simulink model "with_extended_look_ahead"  (R2022a)
settings: Solver=FixedStepAuto  StartTime=0.0  StopTime=18  FixedStep=0.01  RelTol=1e-3
settings Model: Creator=11913  LastModifiedBy=11913

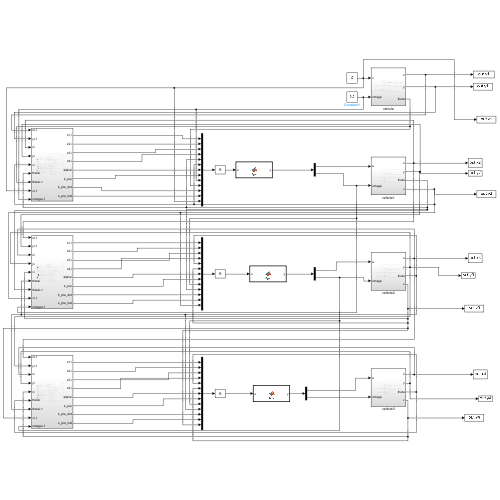
[thumbnail: Simulink's stored preview of the top-level diagram]
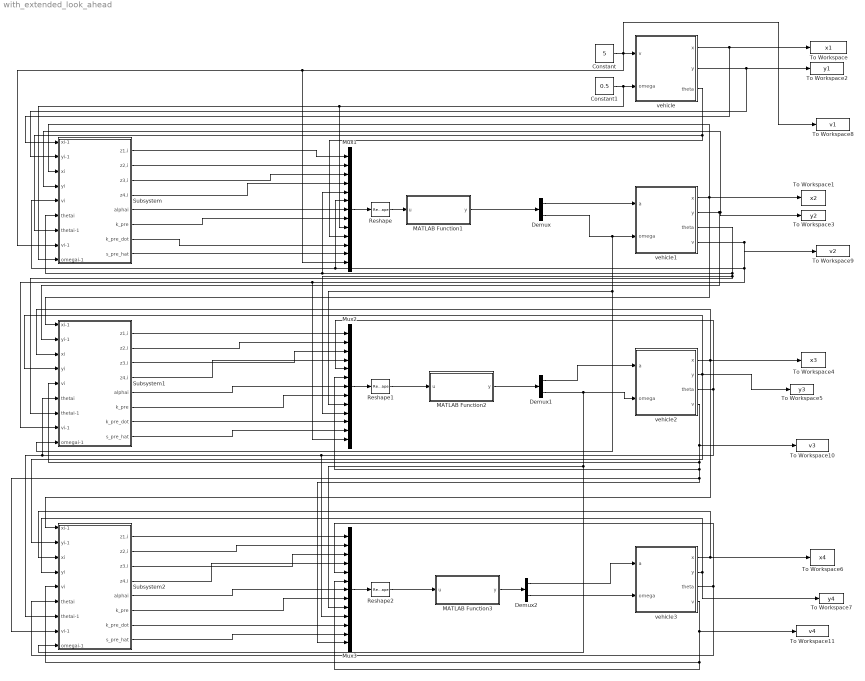
== system with_extended_look_ahead ==
  Constant : Constant  Value=5
  Constant1 : Constant  Value=0.5
  Demux : Demux  Outputs=2
  Demux1 : Demux  Outputs=2
  Demux2 : Demux  Outputs=2
  MATLAB Function1 : MATLAB Function  TreatAsAtomicUnit=on
  MATLAB Function2 : MATLAB Function  TreatAsAtomicUnit=on
  MATLAB Function3 : MATLAB Function  TreatAsAtomicUnit=on
  Mux1 : Mux  Inputs=13
  Mux2 : Mux  Inputs=13
  Mux3 : Mux  Inputs=13
  Reshape : Reshape  OutputDimensionality=Customize  OutputDimensions=[1,13]
  Reshape1 : Reshape  OutputDimensionality=Customize  OutputDimensions=[1,13]
  Reshape2 : Reshape  OutputDimensionality=Customize  OutputDimensions=[1,13]
  Subsystem : Subsystem
  Subsystem1 : Subsystem
  Subsystem2 : Subsystem
  To Workspace : ToWorkspace  VariableName=x1  SampleTime=-1
      settings: Save2DSignal=2-D array (concatenate along first dimension)
  To Workspace1 : ToWorkspace  VariableName=x2  SampleTime=-1
      settings: Save2DSignal=2-D array (concatenate along first dimension)
  To Workspace10 : ToWorkspace  VariableName=v3  SaveFormat=Timeseries  SampleTime=-1
      settings: Save2DSignal=2-D array (concatenate along first dimension)
  To Workspace11 : ToWorkspace  VariableName=v4  SaveFormat=Timeseries  SampleTime=-1
      settings: Save2DSignal=2-D array (concatenate along first dimension)
  To Workspace2 : ToWorkspace  VariableName=y1  SampleTime=-1
      settings: Save2DSignal=2-D array (concatenate along first dimension)
  To Workspace3 : ToWorkspace  VariableName=y2  SampleTime=-1
      settings: Save2DSignal=2-D array (concatenate along first dimension)
  To Workspace4 : ToWorkspace  VariableName=x3  SampleTime=-1
      settings: Save2DSignal=2-D array (concatenate along first dimension)
  To Workspace5 : ToWorkspace  VariableName=y3  SampleTime=-1
      settings: Save2DSignal=2-D array (concatenate along first dimension)
  To Workspace6 : ToWorkspace  VariableName=x4  SampleTime=-1
      settings: Save2DSignal=2-D array (concatenate along first dimension)
  To Workspace7 : ToWorkspace  VariableName=y4  SampleTime=-1
      settings: Save2DSignal=2-D array (concatenate along first dimension)
  To Workspace8 : ToWorkspace  VariableName=v1  SaveFormat=Timeseries  SampleTime=-1
      settings: Save2DSignal=2-D array (concatenate along first dimension)
  To Workspace9 : ToWorkspace  VariableName=v2  SaveFormat=Timeseries  SampleTime=-1
      settings: Save2DSignal=2-D array (concatenate along first dimension)
  vehicle : Subsystem
  vehicle1 : Subsystem
  vehicle2 : Subsystem
  vehicle3 : Subsystem
  wires:
  Constant/1 -> To Workspace8/1, Mux1/13, Subsystem/8(vi-1), vehicle/1(v)
  Constant1/1 -> Subsystem/9(omegai-1), Mux1/9, vehicle/2(omega)
  vehicle/2(y) -> To Workspace2/1, Subsystem/2(yi-1)
  vehicle/1(x) -> To Workspace/1, Subsystem/1(xi-1)
  vehicle/3(theta) -> Mux1/10, Subsystem/7(thetai-1)
  vehicle1/1(x) -> Subsystem1/1(xi-1), Subsystem/3(xi), To Workspace1/1
  vehicle1/2(y) -> Subsystem1/2(yi-1), To Workspace3/1, Subsystem/4(yi)
  vehicle1/4(v) -> To Workspace9/1, Mux2/13, Subsystem1/8(vi-1), Subsystem/5(vi), Mux1/6
  vehicle1/3(theta) -> Mux2/10, Subsystem1/7(thetai-1), Subsystem/6(thetai), Mux1/5
  Subsystem/1(z1,i) -> Mux1/1
  Subsystem/2(z2,i) -> Mux1/2
  Subsystem/3(z3,i) -> Mux1/3
  Subsystem/4(z4,i) -> Mux1/4
  Subsystem/5(alphai) -> Mux1/7
  Subsystem/6(k_pre) -> Mux1/8
  Subsystem/7(k_pre_dot) -> Mux1/11
  Subsystem/8(s_pre_hat) -> Mux1/12
  MATLAB Function1/1(y) -> Demux/1
  Demux/1 -> vehicle1/1(a)
  Demux/2 -> Mux2/9, Subsystem1/9(omegai-1), vehicle1/2(omega)
  Mux1/1 -> Reshape/1
  Reshape/1 -> MATLAB Function1/1(u)
  vehicle2/1(x) -> Subsystem2/1(xi-1), To Workspace4/1, Subsystem1/3(xi)
  vehicle2/2(y) -> Subsystem2/2(yi-1), To Workspace5/1, Subsystem1/4(yi)
  vehicle2/4(v) -> To Workspace10/1, Mux3/13, Subsystem2/8(vi-1), Mux2/6, Subsystem1/5(vi)
  vehicle2/3(theta) -> Mux3/10, Subsystem2/7(thetai-1), Subsystem1/6(thetai), Mux2/5
  Subsystem1/1(z1,i) -> Mux2/1
  Subsystem1/2(z2,i) -> Mux2/2
  Subsystem1/3(z3,i) -> Mux2/3
  Subsystem1/4(z4,i) -> Mux2/4
  Subsystem1/5(alphai) -> Mux2/7
  Subsystem1/6(k_pre) -> Mux2/8
  Subsystem1/7(k_pre_dot) -> Mux2/11
  Subsystem1/8(s_pre_hat) -> Mux2/12
  Mux2/1 -> Reshape1/1
  Reshape1/1 -> MATLAB Function2/1(u)
  MATLAB Function2/1(y) -> Demux1/1
  Demux1/1 -> vehicle2/1(a)
  Demux1/2 -> Mux3/9, Subsystem2/9(omegai-1), vehicle2/2(omega)
  vehicle3/1(x) -> To Workspace6/1, Subsystem2/3(xi)
  vehicle3/2(y) -> To Workspace7/1, Subsystem2/4(yi)
  vehicle3/4(v) -> Mux3/6, Subsystem2/5(vi), To Workspace11/1
  vehicle3/3(theta) -> Subsystem2/6(thetai), Mux3/5
  Subsystem2/1(z1,i) -> Mux3/1
  Subsystem2/2(z2,i) -> Mux3/2
  Subsystem2/3(z3,i) -> Mux3/3
  Subsystem2/4(z4,i) -> Mux3/4
  Subsystem2/5(alphai) -> Mux3/7
  Subsystem2/6(k_pre) -> Mux3/8
  Subsystem2/7(k_pre_dot) -> Mux3/11
  Subsystem2/8(s_pre_hat) -> Mux3/12
  Mux3/1 -> Reshape2/1
  Reshape2/1 -> MATLAB Function3/1(u)
  MATLAB Function3/1(y) -> Demux2/1
  Demux2/1 -> vehicle3/1(a)
  Demux2/2 -> vehicle3/2(omega)

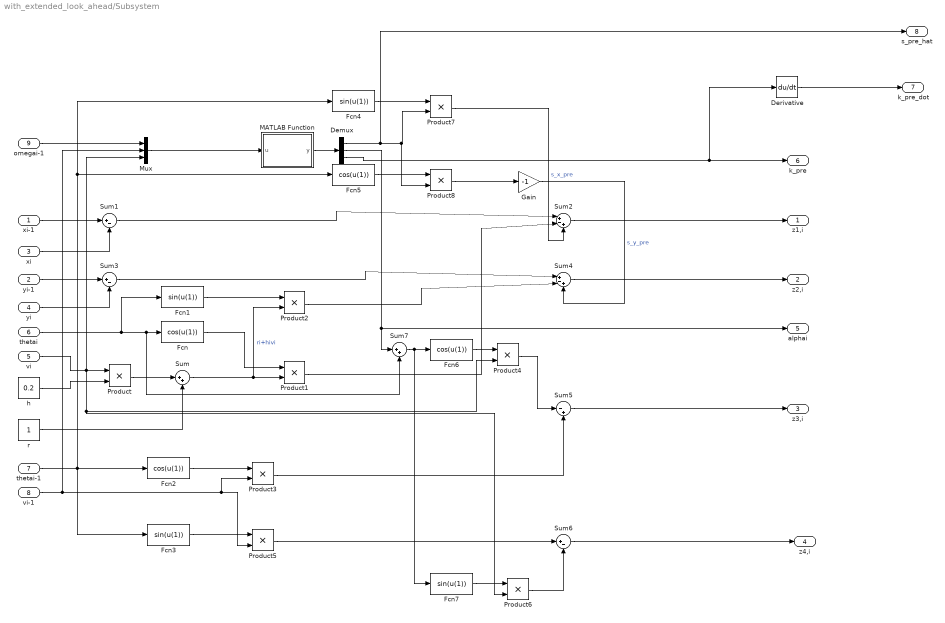
== system with_extended_look_ahead/Subsystem ==
  xi-1 : Inport
  yi-1 : Inport  Port=2
  xi : Inport  Port=3
  yi : Inport  Port=4
  vi : Inport  Port=5
  thetai : Inport  Port=6
  thetai-1 : Inport  Port=7
  vi-1 : Inport  Port=8
  omegai-1 : Inport  Port=9
  Demux : Demux  Outputs=3
  Derivative : Derivative
  Fcn{,2,5..6} (4 alike) : Fcn  Expr=cos(u(1))
  Fcn{1,3..4,7} (4 alike) : Fcn  Expr=sin(u(1))
  Gain : Gain  Gain=-1
  MATLAB Function : MATLAB Function  TreatAsAtomicUnit=on
  Mux : Mux  Inputs=3
  Product{,1..8} (9 alike) : Product
  Sum : Sum  Inputs=|++
  Sum1 : Sum  Inputs=|+-
  Sum2 : Sum  Inputs=|+-+
  Sum3 : Sum  Inputs=|+-
  Sum4 : Sum  Inputs=|+-+
  Sum5 : Sum  Inputs=|-+
  Sum6 : Sum  Inputs=|+-
  Sum7 : Sum  Inputs=|++
  h : Constant  Value=0.2
  r : Constant
  z1,i : Outport
  z2,i : Outport  Port=2
  z3,i : Outport  Port=3
  z4,i : Outport  Port=4
  alphai : Outport  Port=5
  k_pre : Outport  Port=6
  k_pre_dot : Outport  Port=7
  s_pre_hat : Outport  Port=8
  wires:
  vi/1 -> Product6/2, Product4/2, Mux/3, Product/1
  h/1 -> Product/2
  Product/1 -> Sum/1
  r/1 -> Sum/2
  xi-1/1 -> Sum1/1
  xi/1 -> Sum1/2
  thetai/1 -> Sum7/2, Fcn/1, Fcn1/1
  Sum/1 -> Product2/2, Product1/2  "ri+hivi"
  Fcn/1 -> Product1/1
  Sum1/1 -> Sum2/1
  Product1/1 -> Sum2/2
  yi-1/1 -> Sum3/1
  yi/1 -> Sum3/2
  Fcn1/1 -> Product2/1
  Sum3/1 -> Sum4/1
  Product2/1 -> Sum4/2
  Sum4/1 -> z2,i/1
  Sum2/1 -> z1,i/1
  thetai-1/1 -> Fcn5/1, Fcn4/1, Fcn3/1, Fcn2/1
  Fcn2/1 -> Product3/1
  vi-1/1 -> Mux/2, Product5/2, Product3/2
  Product3/1 -> Sum5/2
  Sum5/1 -> z3,i/1
  Fcn3/1 -> Product5/1
  Product5/1 -> Sum6/1
  Sum6/1 -> z4,i/1
  omegai-1/1 -> Mux/1
  Mux/1 -> MATLAB Function/1(u)
  Fcn4/1 -> Product7/1
  Product7/1 -> Sum2/3  "s_x_pre"
  Fcn5/1 -> Product8/1
  Product8/1 -> Gain/1
  Gain/1 -> Sum4/3  "s_y_pre"
  MATLAB Function/1(y) -> Demux/1
  Demux/1 -> s_pre_hat/1, Product8/2, Product7/2
  Demux/2 -> alphai/1, Sum7/1
  Sum7/1 -> Fcn7/1, Fcn6/1
  Fcn6/1 -> Product4/1
  Product4/1 -> Sum5/1
  Fcn7/1 -> Product6/1
  Product6/1 -> Sum6/2
  Demux/3 -> Derivative/1, k_pre/1
  Derivative/1 -> k_pre_dot/1

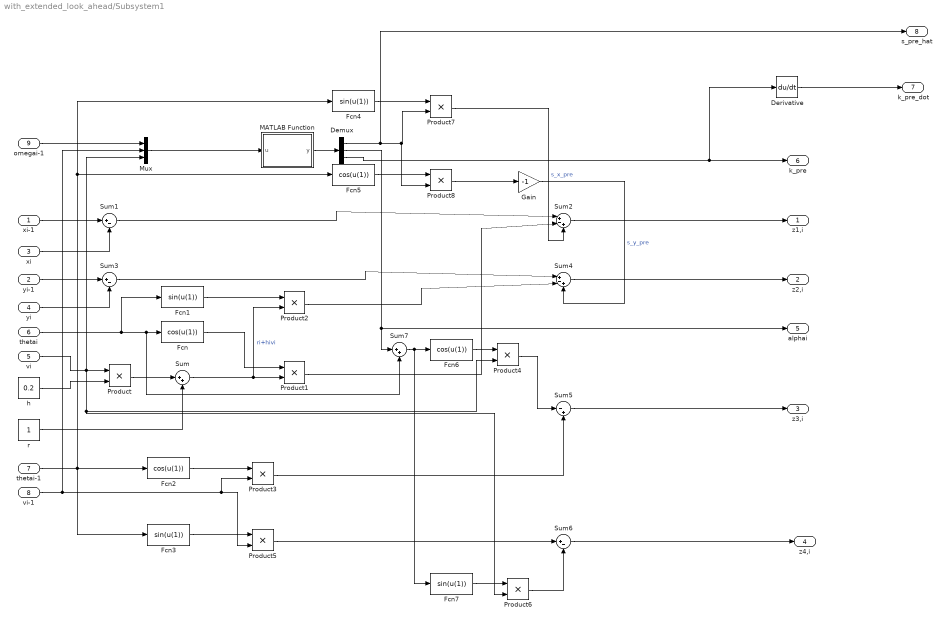
== system with_extended_look_ahead/Subsystem1 ==
  xi-1 : Inport
  yi-1 : Inport  Port=2
  xi : Inport  Port=3
  yi : Inport  Port=4
  vi : Inport  Port=5
  thetai : Inport  Port=6
  thetai-1 : Inport  Port=7
  vi-1 : Inport  Port=8
  omegai-1 : Inport  Port=9
  Demux : Demux  Outputs=3
  Derivative : Derivative
  Fcn{,2,5..6} (4 alike) : Fcn  Expr=cos(u(1))
  Fcn{1,3..4,7} (4 alike) : Fcn  Expr=sin(u(1))
  Gain : Gain  Gain=-1
  MATLAB Function : MATLAB Function  TreatAsAtomicUnit=on
  Mux : Mux  Inputs=3
  Product{,1..8} (9 alike) : Product
  Sum : Sum  Inputs=|++
  Sum1 : Sum  Inputs=|+-
  Sum2 : Sum  Inputs=|+-+
  Sum3 : Sum  Inputs=|+-
  Sum4 : Sum  Inputs=|+-+
  Sum5 : Sum  Inputs=|-+
  Sum6 : Sum  Inputs=|+-
  Sum7 : Sum  Inputs=|++
  h : Constant  Value=0.2
  r : Constant
  z1,i : Outport
  z2,i : Outport  Port=2
  z3,i : Outport  Port=3
  z4,i : Outport  Port=4
  alphai : Outport  Port=5
  k_pre : Outport  Port=6
  k_pre_dot : Outport  Port=7
  s_pre_hat : Outport  Port=8
  wires:
  vi/1 -> Product6/2, Product4/2, Mux/3, Product/1
  h/1 -> Product/2
  Product/1 -> Sum/1
  r/1 -> Sum/2
  xi-1/1 -> Sum1/1
  xi/1 -> Sum1/2
  thetai/1 -> Sum7/2, Fcn/1, Fcn1/1
  Sum/1 -> Product2/2, Product1/2  "ri+hivi"
  Fcn/1 -> Product1/1
  Sum1/1 -> Sum2/1
  Product1/1 -> Sum2/2
  yi-1/1 -> Sum3/1
  yi/1 -> Sum3/2
  Fcn1/1 -> Product2/1
  Sum3/1 -> Sum4/1
  Product2/1 -> Sum4/2
  Sum4/1 -> z2,i/1
  Sum2/1 -> z1,i/1
  thetai-1/1 -> Fcn5/1, Fcn4/1, Fcn3/1, Fcn2/1
  Fcn2/1 -> Product3/1
  vi-1/1 -> Mux/2, Product5/2, Product3/2
  Product3/1 -> Sum5/2
  Sum5/1 -> z3,i/1
  Fcn3/1 -> Product5/1
  Product5/1 -> Sum6/1
  Sum6/1 -> z4,i/1
  omegai-1/1 -> Mux/1
  Mux/1 -> MATLAB Function/1(u)
  Fcn4/1 -> Product7/1
  Product7/1 -> Sum2/3  "s_x_pre"
  Fcn5/1 -> Product8/1
  Product8/1 -> Gain/1
  Gain/1 -> Sum4/3  "s_y_pre"
  MATLAB Function/1(y) -> Demux/1
  Demux/1 -> s_pre_hat/1, Product8/2, Product7/2
  Demux/2 -> alphai/1, Sum7/1
  Sum7/1 -> Fcn7/1, Fcn6/1
  Fcn6/1 -> Product4/1
  Product4/1 -> Sum5/1
  Fcn7/1 -> Product6/1
  Product6/1 -> Sum6/2
  Demux/3 -> Derivative/1, k_pre/1
  Derivative/1 -> k_pre_dot/1

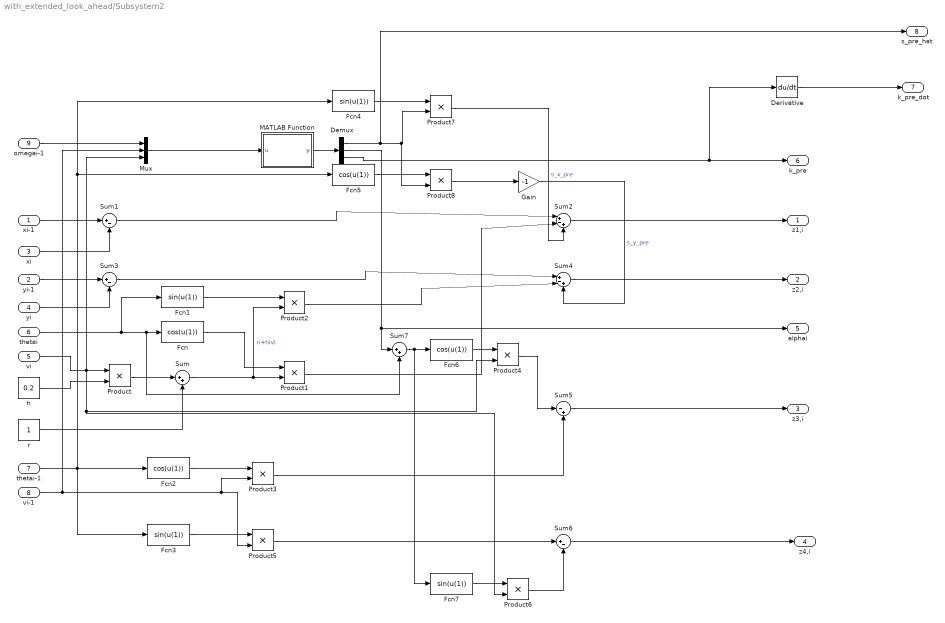
== system with_extended_look_ahead/Subsystem2 ==
  xi-1 : Inport
  yi-1 : Inport  Port=2
  xi : Inport  Port=3
  yi : Inport  Port=4
  vi : Inport  Port=5
  thetai : Inport  Port=6
  thetai-1 : Inport  Port=7
  vi-1 : Inport  Port=8
  omegai-1 : Inport  Port=9
  Demux : Demux  Outputs=3
  Derivative : Derivative
  Fcn{,2,5..6} (4 alike) : Fcn  Expr=cos(u(1))
  Fcn{1,3..4,7} (4 alike) : Fcn  Expr=sin(u(1))
  Gain : Gain  Gain=-1
  MATLAB Function : MATLAB Function  TreatAsAtomicUnit=on
  Mux : Mux  Inputs=3
  Product{,1..8} (9 alike) : Product
  Sum : Sum  Inputs=|++
  Sum1 : Sum  Inputs=|+-
  Sum2 : Sum  Inputs=|+-+
  Sum3 : Sum  Inputs=|+-
  Sum4 : Sum  Inputs=|+-+
  Sum5 : Sum  Inputs=|-+
  Sum6 : Sum  Inputs=|+-
  Sum7 : Sum  Inputs=|++
  h : Constant  Value=0.2
  r : Constant
  z1,i : Outport
  z2,i : Outport  Port=2
  z3,i : Outport  Port=3
  z4,i : Outport  Port=4
  alphai : Outport  Port=5
  k_pre : Outport  Port=6
  k_pre_dot : Outport  Port=7
  s_pre_hat : Outport  Port=8
  wires:
  vi/1 -> Product6/2, Product4/2, Mux/3, Product/1
  h/1 -> Product/2
  Product/1 -> Sum/1
  r/1 -> Sum/2
  xi-1/1 -> Sum1/1
  xi/1 -> Sum1/2
  thetai/1 -> Sum7/2, Fcn/1, Fcn1/1
  Sum/1 -> Product2/2, Product1/2  "ri+hivi"
  Fcn/1 -> Product1/1
  Sum1/1 -> Sum2/1
  Product1/1 -> Sum2/2
  yi-1/1 -> Sum3/1
  yi/1 -> Sum3/2
  Fcn1/1 -> Product2/1
  Sum3/1 -> Sum4/1
  Product2/1 -> Sum4/2
  Sum4/1 -> z2,i/1
  Sum2/1 -> z1,i/1
  thetai-1/1 -> Fcn5/1, Fcn4/1, Fcn3/1, Fcn2/1
  Fcn2/1 -> Product3/1
  vi-1/1 -> Mux/2, Product5/2, Product3/2
  Product3/1 -> Sum5/2
  Sum5/1 -> z3,i/1
  Fcn3/1 -> Product5/1
  Product5/1 -> Sum6/1
  Sum6/1 -> z4,i/1
  omegai-1/1 -> Mux/1
  Mux/1 -> MATLAB Function/1(u)
  Fcn4/1 -> Product7/1
  Product7/1 -> Sum2/3  "s_x_pre"
  Fcn5/1 -> Product8/1
  Product8/1 -> Gain/1
  Gain/1 -> Sum4/3  "s_y_pre"
  MATLAB Function/1(y) -> Demux/1
  Demux/1 -> s_pre_hat/1, Product8/2, Product7/2
  Demux/2 -> alphai/1, Sum7/1
  Sum7/1 -> Fcn7/1, Fcn6/1
  Fcn6/1 -> Product4/1
  Product4/1 -> Sum5/1
  Fcn7/1 -> Product6/1
  Product6/1 -> Sum6/2
  Demux/3 -> Derivative/1, k_pre/1
  Derivative/1 -> k_pre_dot/1

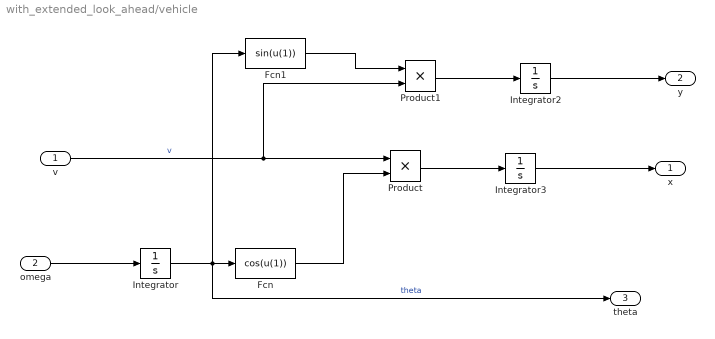
== system with_extended_look_ahead/vehicle ==
  v : Inport
  omega : Inport  Port=2
  Fcn : Fcn  Expr=cos(u(1))
  Fcn1 : Fcn  Expr=sin(u(1))
  Integrator : Integrator
  Integrator2 : Integrator
  Integrator3 : Integrator
  Product : Product
  Product1 : Product
  x : Outport
  y : Outport  Port=2
  theta : Outport  Port=3
  wires:
  omega/1 -> Integrator/1
  Integrator/1 -> theta/1, Fcn1/1, Fcn/1  "theta"
  v/1 -> Product1/2, Product/1  "v"
  Fcn/1 -> Product/2
  Fcn1/1 -> Product1/1
  Product1/1 -> Integrator2/1
  Product/1 -> Integrator3/1
  Integrator2/1 -> y/1
  Integrator3/1 -> x/1

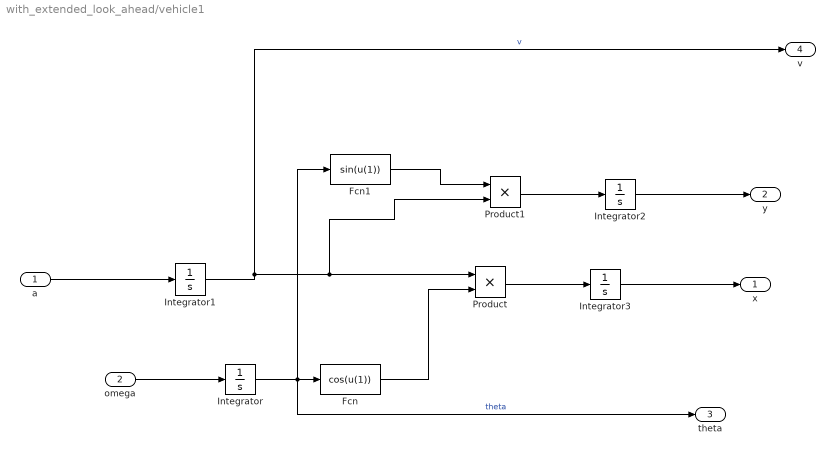
== system with_extended_look_ahead/vehicle1 ==
  a : Inport
  omega : Inport  Port=2
  Fcn : Fcn  Expr=cos(u(1))
  Fcn1 : Fcn  Expr=sin(u(1))
  Integrator : Integrator
  Integrator1 : Integrator  InitialCondition=5  LowerSaturationLimit=0
  Integrator2 : Integrator  InitialCondition=2
  Integrator3 : Integrator  InitialCondition=-2
  Product : Product
  Product1 : Product
  x : Outport
  y : Outport  Port=2
  theta : Outport  Port=3
  v : Outport  Port=4
  wires:
  omega/1 -> Integrator/1
  Integrator/1 -> theta/1, Fcn1/1, Fcn/1  "theta"
  Fcn/1 -> Product/2
  Fcn1/1 -> Product1/1
  Product1/1 -> Integrator2/1
  Product/1 -> Integrator3/1
  Integrator2/1 -> y/1
  Integrator3/1 -> x/1
  a/1 -> Integrator1/1
  Integrator1/1 -> v/1, Product1/2, Product/1  "v"

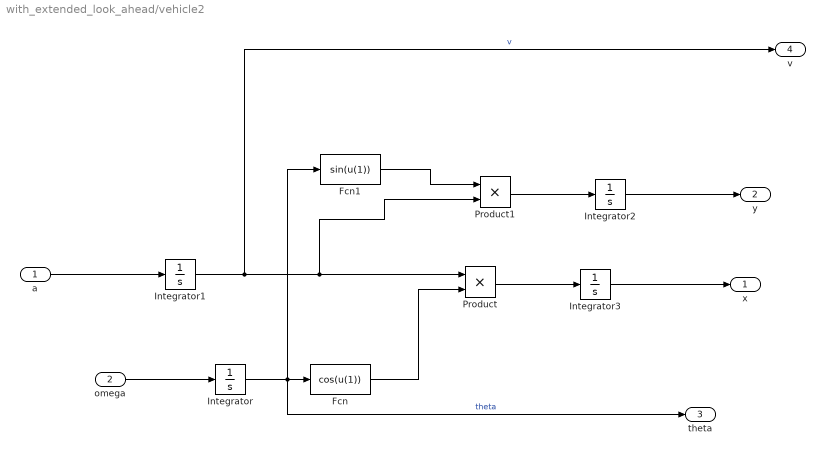
== system with_extended_look_ahead/vehicle2 ==
  a : Inport
  omega : Inport  Port=2
  Fcn : Fcn  Expr=cos(u(1))
  Fcn1 : Fcn  Expr=sin(u(1))
  Integrator : Integrator
  Integrator1 : Integrator  InitialCondition=5
  Integrator2 : Integrator  InitialCondition=4
  Integrator3 : Integrator  InitialCondition=-4
  Product : Product
  Product1 : Product
  x : Outport
  y : Outport  Port=2
  theta : Outport  Port=3
  v : Outport  Port=4
  wires:
  omega/1 -> Integrator/1
  Integrator/1 -> theta/1, Fcn1/1, Fcn/1  "theta"
  Fcn/1 -> Product/2
  Fcn1/1 -> Product1/1
  Product1/1 -> Integrator2/1
  Product/1 -> Integrator3/1
  Integrator2/1 -> y/1
  Integrator3/1 -> x/1
  a/1 -> Integrator1/1
  Integrator1/1 -> v/1, Product1/2, Product/1  "v"

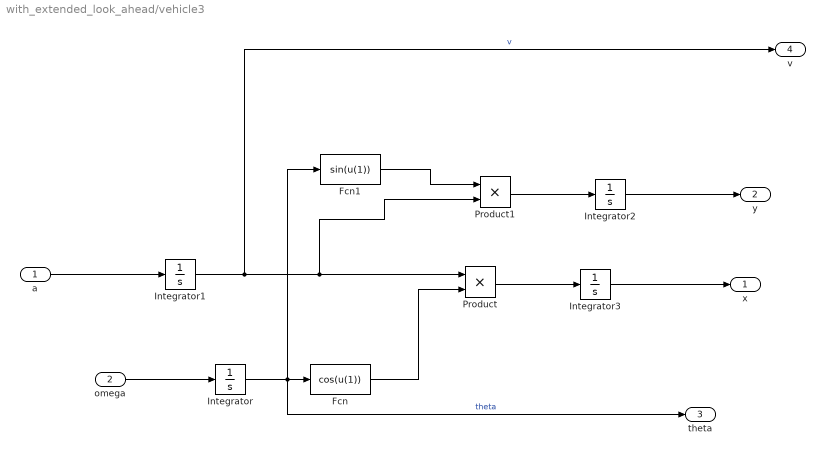
== system with_extended_look_ahead/vehicle3 ==
  a : Inport
  omega : Inport  Port=2
  Fcn : Fcn  Expr=cos(u(1))
  Fcn1 : Fcn  Expr=sin(u(1))
  Integrator : Integrator
  Integrator1 : Integrator  InitialCondition=5
  Integrator2 : Integrator  InitialCondition=6
  Integrator3 : Integrator  InitialCondition=-6
  Product : Product
  Product1 : Product
  x : Outport
  y : Outport  Port=2
  theta : Outport  Port=3
  v : Outport  Port=4
  wires:
  omega/1 -> Integrator/1
  Integrator/1 -> theta/1, Fcn1/1, Fcn/1  "theta"
  Fcn/1 -> Product/2
  Fcn1/1 -> Product1/1
  Product1/1 -> Integrator2/1
  Product/1 -> Integrator3/1
  Integrator2/1 -> y/1
  Integrator3/1 -> x/1
  a/1 -> Integrator1/1
  Integrator1/1 -> v/1, Product1/2, Product/1  "v"

== matlab function with_extended_look_ahead/Subsystem1/MATLAB Function ==
  data: u input; y output
function y = fcn(u)
r=1;
h=0.2;
omega_pre=u(1);
v_pre=u(2);
vi=u(3);
k_pre=omega_pre/v_pre;
if k_pre==0
    s_pre_hat=0;
else
    s_pre_hat=(sqrt(1+k_pre^2*(r+h*vi)^2)-1)/k_pre;
end

alphai=atan(k_pre*(r+h*vi));
y = [s_pre_hat;alphai;k_pre];

== matlab function with_extended_look_ahead/MATLAB Function2 ==
  data: u input; y output
function y = fcn(u)
z1_i=u(1);
z2_i=u(2);
z3_i=u(3);
z4_i=u(4);
thetai=u(5);
vi=u(6);
alphai=u(7);
k_pre=u(8);
omegai_pre=u(9);
thetai_pre=u(10);
k_pre_dot=u(11);
s_pre_hat=u(12);
vi_pre=u(13);

k1=3.5;
k2=3.5;
r=1;
h=0.2;

%计算β1,i；
if k_pre==0
    ski=0;
else
    ski=(1/(k_pre)^2)*(1-cos(alphai));
end
R_theta_pre=[cos(thetai_pre),-sin(thetai_pre);sin(thetai_pre),cos(thetai_pre)];
beta1i=[-sin(thetai);cos(thetai)]*vi*tan(alphai)+R_theta_pre*[s_pre_hat*omegai_pre;-ski*k_pre_dot]+(1-1/cos(alphai))*[cos(thetai_pre);sin(thetai_pre)]*vi_pre;

%计算前面那个矩阵
sai=h*sin(alphai);
miui=h*(r+h*vi)*(1-sin(alphai)*sin(thetai_pre-thetai));
F_inv_11=(r+h*vi)*cos(thetai);
F_inv_12=(r+h*vi)*sin(thetai);
F_inv_21=-h*sin(thetai)-sai*cos(thetai_pre);
F_inv_22=h*cos(thetai)-sai*sin(thetai_pre);
T_inv=(1/miui)*[F_inv_11,F_inv_12;F_inv_21,F_inv_22];

%计算输入矩阵[α，ω]
result=T_inv*([k1*z1_i;k2*z2_i]+(1/cos(alphai))*[z3_i;z4_i]+beta1i);



y = result;

== matlab function with_extended_look_ahead/Subsystem/MATLAB Function ==
  data: u input; y output
function y = fcn(u)
r=1;
h=0.2;
omega_pre=u(1);
v_pre=u(2);
vi=u(3);
k_pre=omega_pre/v_pre;
if k_pre==0
    s_pre_hat=0;
else
    s_pre_hat=(sqrt(1+k_pre^2*(r+h*vi)^2)-1)/k_pre;
end

alphai=atan(k_pre*(r+h*vi));
y = [s_pre_hat;alphai;k_pre];

== matlab function with_extended_look_ahead/Subsystem2/MATLAB Function ==
  data: u input; y output
function y = fcn(u)
r=1;
h=0.2;
omega_pre=u(1);
v_pre=u(2);
vi=u(3);
k_pre=omega_pre/v_pre;
if k_pre==0
    s_pre_hat=0;
else
    s_pre_hat=(sqrt(1+k_pre^2*(r+h*vi)^2)-1)/k_pre;
end

alphai=atan(k_pre*(r+h*vi));
y = [s_pre_hat;alphai;k_pre];

== matlab function with_extended_look_ahead/MATLAB Function3 ==
  data: u input; y output
function y = fcn(u)
z1_i=u(1);
z2_i=u(2);
z3_i=u(3);
z4_i=u(4);
thetai=u(5);
vi=u(6);
alphai=u(7);
k_pre=u(8);
omegai_pre=u(9);
thetai_pre=u(10);
k_pre_dot=u(11);
s_pre_hat=u(12);
vi_pre=u(13);

k1=3.5;
k2=3.5;
r=1;
h=0.2;

%计算β1,i；
if k_pre==0
    ski=0;
else
    ski=(1/(k_pre)^2)*(1-cos(alphai));
end
R_theta_pre=[cos(thetai_pre),-sin(thetai_pre);sin(thetai_pre),cos(thetai_pre)];
beta1i=[-sin(thetai);cos(thetai)]*vi*tan(alphai)+R_theta_pre*[s_pre_hat*omegai_pre;-ski*k_pre_dot]+(1-1/cos(alphai))*[cos(thetai_pre);sin(thetai_pre)]*vi_pre;

%计算前面那个矩阵
sai=h*sin(alphai);
miui=h*(r+h*vi)*(1-sin(alphai)*sin(thetai_pre-thetai));
F_inv_11=(r+h*vi)*cos(thetai);
F_inv_12=(r+h*vi)*sin(thetai);
F_inv_21=-h*sin(thetai)-sai*cos(thetai_pre);
F_inv_22=h*cos(thetai)-sai*sin(thetai_pre);
T_inv=(1/miui)*[F_inv_11,F_inv_12;F_inv_21,F_inv_22];

%计算输入矩阵[α，ω]
result=T_inv*([k1*z1_i;k2*z2_i]+(1/cos(alphai))*[z3_i;z4_i]+beta1i);



y = result;

== matlab function with_extended_look_ahead/MATLAB Function1 ==
  data: u input; y output
function y = fcn(u)
z1_i=u(1);
z2_i=u(2);
z3_i=u(3);
z4_i=u(4);
thetai=u(5);
vi=u(6);
alphai=u(7);
k_pre=u(8);
omegai_pre=u(9);
thetai_pre=u(10);
k_pre_dot=u(11);
s_pre_hat=u(12);
vi_pre=u(13);

k1=3.5;
k2=3.5;
r=1;
h=0.2;

%计算β1,i；
if k_pre==0
    ski=0;
else
    ski=(1/(k_pre)^2)*(1-cos(alphai));
end
R_theta_pre=[cos(thetai_pre),-sin(thetai_pre);sin(thetai_pre),cos(thetai_pre)];
beta1i=[-sin(thetai);cos(thetai)]*vi*tan(alphai)+R_theta_pre*[s_pre_hat*omegai_pre;-ski*k_pre_dot]+(1-1/cos(alphai))*[cos(thetai_pre);sin(thetai_pre)]*vi_pre;

%计算前面那个矩阵
sai=h*sin(alphai);
miui=h*(r+h*vi)*(1-sin(alphai)*sin(thetai_pre-thetai));
F_inv_11=(r+h*vi)*cos(thetai);
F_inv_12=(r+h*vi)*sin(thetai);
F_inv_21=-h*sin(thetai)-sai*cos(thetai_pre);
F_inv_22=h*cos(thetai)-sai*sin(thetai_pre);
T_inv=(1/miui)*[F_inv_11,F_inv_12;F_inv_21,F_inv_22];

%计算输入矩阵[α，ω]
result=T_inv*([k1*z1_i;k2*z2_i]+(1/cos(alphai))*[z3_i;z4_i]+beta1i);



y = result;
